simulink model "Q2_4"  (R2021b)
settings: Solver=VariableStepAuto  StartTime=0.0  StopTime=10.0  RelTol=1e-3
values from neighbouring files (symbols this model uses):
  CA0 = 10    [Q2_4_DATA.m]
  p0 = 3+F/V    (= 3.52631578947)    [Q2_4_DATA.m]
  p1 = F/V    (= 0.526315789474)    [Q2_4_DATA.m]
  t0 = CA0*F/V    (= 5.26315789474)    [Q2_4_DATA.m]
  t1 = F/V*Tf+Og/(Cp*rou*V)    (= 131.579013158)    [Q2_4_DATA.m]
  Tf = 250    [Q2_4_DATA.m]
settings Model: Creator=Sinon  LastModifiedBy=Sinon

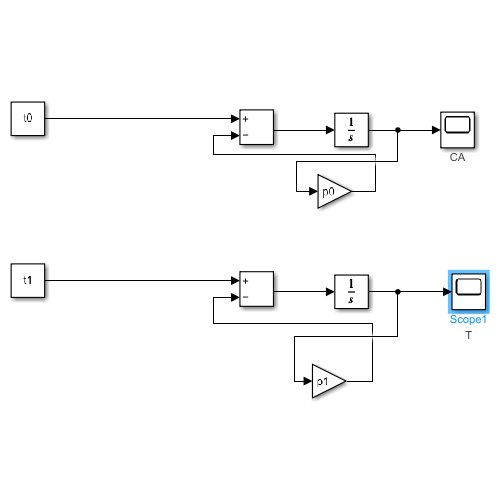
[thumbnail: Simulink's stored preview of the top-level diagram]
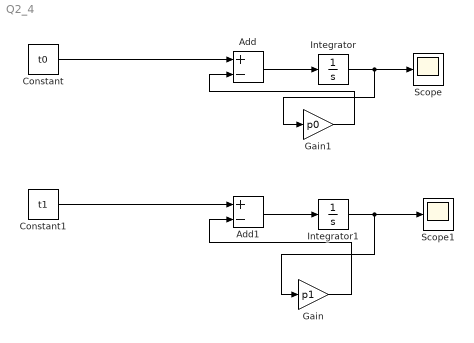
== system Q2_4 ==
  Add : Sum  Inputs=+-
  Add1 : Sum  Inputs=+-
  Constant : Constant  Value=t0
  Constant1 : Constant  Value=t1
  Gain : Gain  Gain=p1
  Gain1 : Gain  Gain=p0
  Integrator : Integrator  InitialCondition=CA0
  Integrator1 : Integrator  InitialCondition=Tf
  Scope : Scope
      settings: AttributesFormatString=CA
  Scope1 : Scope
      settings: AttributesFormatString=T
  wires:
  Integrator/1 -> Gain1/1, Scope/1
  Add/1 -> Integrator/1
  Gain1/1 -> Add/2
  Constant/1 -> Add/1
  Add1/1 -> Integrator1/1
  Integrator1/1 -> Gain/1, Scope1/1
  Gain/1 -> Add1/2
  Constant1/1 -> Add1/1
